simulink model "DeadTimevsTimeConstant"  (R2017b)
settings: Solver=VariableStepAuto  StartTime=0.0  StopTime=10.0  RelTol=1e-3
libraries: simulink x1
settings Model: Creator=k37107  LastModifiedBy=k37107

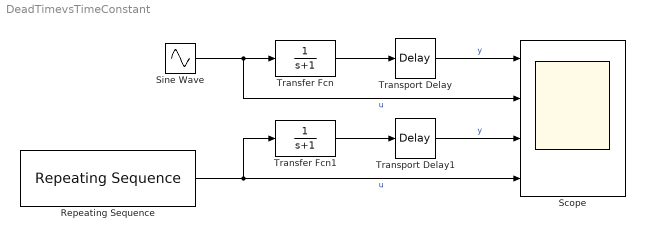
== system DeadTimevsTimeConstant ==
  Repeating Sequence : simulink/Sources/Repeating Sequence  rep_seq_t=[0 pi/2 pi 3/2*pi 2*pi]  rep_seq_y=[0 1 0 -1 0]
  Scope : Scope  NumInputPorts=4
  Sine Wave : Sin  SampleTime=0
  Transfer Fcn : TransferFcn  Denominator=[1 1]
  Transfer Fcn1 : TransferFcn  Denominator=[1 1]
  Transport Delay : TransportDelay
  Transport Delay1 : TransportDelay
  wires:
  Sine Wave/1 -> Transfer Fcn/1, Scope/2  "u"
  Transport Delay/1 -> Scope/1  "y"
  Transfer Fcn/1 -> Transport Delay/1
  Transfer Fcn1/1 -> Transport Delay1/1
  Transport Delay1/1 -> Scope/3  "y"
  Repeating Sequence/1 -> Transfer Fcn1/1, Scope/4  "u"
